simulink model "onearea_SOC"  (R2018b)
settings: Solver=ode3  StartTime=0.0  StopTime=20  FixedStep=0.1  RelTol=1e-3  EnableMultiTasking=on
values from neighbouring files (symbols this model uses):
  fH3 = 61    [oneareaSOC.m]
  fL3 = 59    [oneareaSOC.m]
  Ki = 0.1    [oneareaSOC.m]
  PRi = 0    [oneareaSOC.m]
  R = 3    [oneareaSOC.m]
  SOC = 1    [oneareaSOC.m]
undefined symbols (not defined in the file or in its folder): f
libraries: simulink_need_slupdate x1, simulink x1
settings Model: Creator=EPESL  LastModifiedBy=EPESL
settings DebuggingCC: UnderSpecifiedDimensionMsg=warning

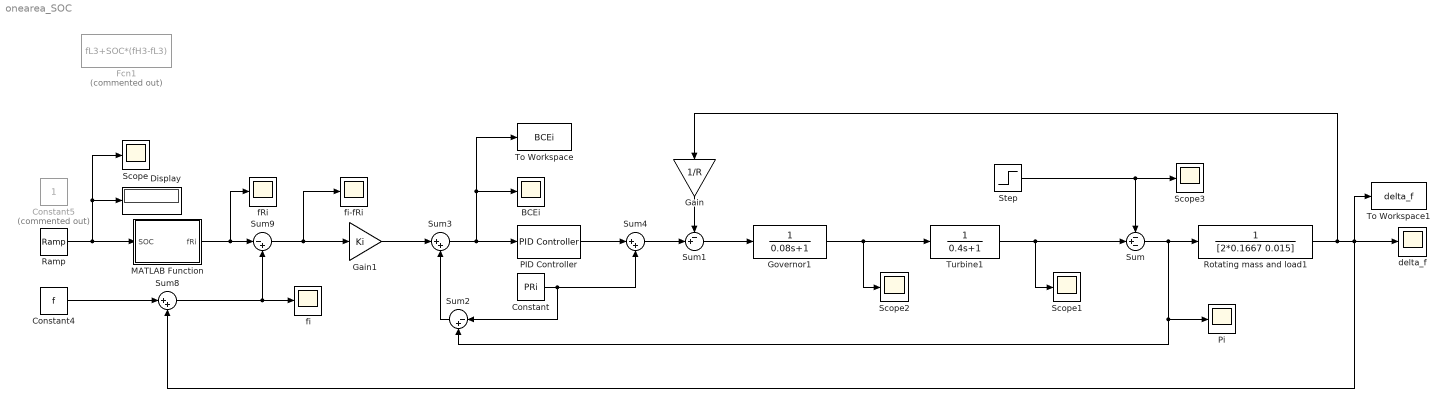
== system onearea_SOC ==
  BCEi : Scope
  Constant : Constant  Value=PRi
  Constant4 : Constant  Value=f
  Constant5 : Constant  Commented=on
  Display : Display
  Fcn1 : Fcn  Commented=on  Expr=fL3+SOC*(fH3-fL3)
  Gain : Gain  Gain=1/R
  Gain1 : Gain  Gain=Ki
  Governor1 : TransferFcn  Denominator=[0.08 1]
  MATLAB Function : MATLAB Function  TreatAsAtomicUnit=on
  PID Controller : simulink_need_slupdate/PID Controller  P=0  I=-0.3  D=0
      settings: SourceProductName=Simulink
  Pi : Scope
  Ramp : simulink/Sources/Ramp  slope=-1/20  start=0  InitialOutput=1
  Rotating mass and load1 : TransferFcn  Denominator=[2*0.1667 0.015]
  Scope{,1..3} (4 alike) : Scope
  Step : Step  Time=0  After=0  SampleTime=0
  Sum : Sum  Inputs=-+-
  Sum1 : Sum  Inputs=-+|
  Sum2 : Sum  Inputs=|-+
  Sum3 : Sum  Inputs=|++
  Sum4 : Sum  Inputs=|++
  Sum8 : Sum  Inputs=|++
  Sum9 : Sum  Inputs=|-+
  To Workspace : ToWorkspace  VariableName=BCEi  SampleTime=-1
  To Workspace1 : ToWorkspace  VariableName=delta_f  SampleTime=-1
  Turbine1 : TransferFcn  Denominator=[0.4 1]
  delta_f : Scope
  fRi : Scope
  fi : Scope
  fi-fRi : Scope
  wires:
  Gain/1 -> Sum1/1
  Step/1 -> Scope3/1, Sum/1
  Constant4/1 -> Sum8/1
  MATLAB Function/1(fRi) -> Sum9/1, fRi/1
  Sum8/1 -> fi/1, Sum9/2
  Sum9/1 -> fi-fRi/1, Gain1/1
  Sum/1 -> Sum2/2, Pi/1, Rotating mass and load1/1
  Rotating mass and load1/1 -> Sum8/2, To Workspace1/1, delta_f/1, Gain/1
  Turbine1/1 -> Scope1/1, Sum/2
  Sum1/1 -> Governor1/1
  Governor1/1 -> Scope2/1, Turbine1/1
  Gain1/1 -> Sum3/1
  Sum3/1 -> BCEi/1, To Workspace/1, PID Controller/1
  Sum2/1 -> Sum3/2
  PID Controller/1 -> Sum4/1
  Sum4/1 -> Sum1/2
  Constant/1 -> Sum4/2, Sum2/1
  Ramp/1 -> MATLAB Function/1(SOC), Scope/1, Display/1

== matlab function onearea_SOC/MATLAB Function ==
  data: SOC input; fRi output
function fRi = Func(SOC)

fRi = 59+SOC*(61-59);
